simulink model "AircraftSim"  (R2025b)
settings: Solver=VariableStepAuto  StartTime=0.0  StopTime=10.0  RelTol=1e-3
libraries: simulink x6
settings Model: Creator=deepa  LastModifiedBy=deepa

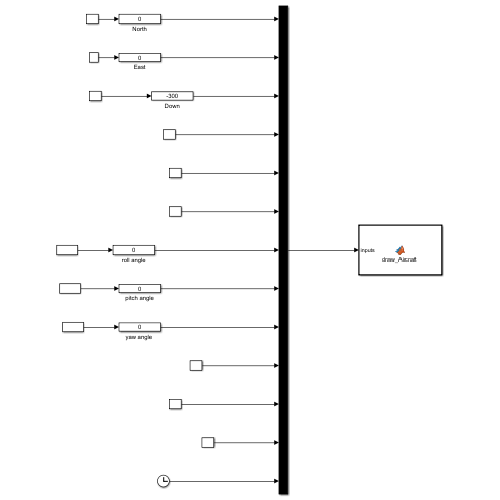
[thumbnail: Simulink's stored preview of the top-level diagram]
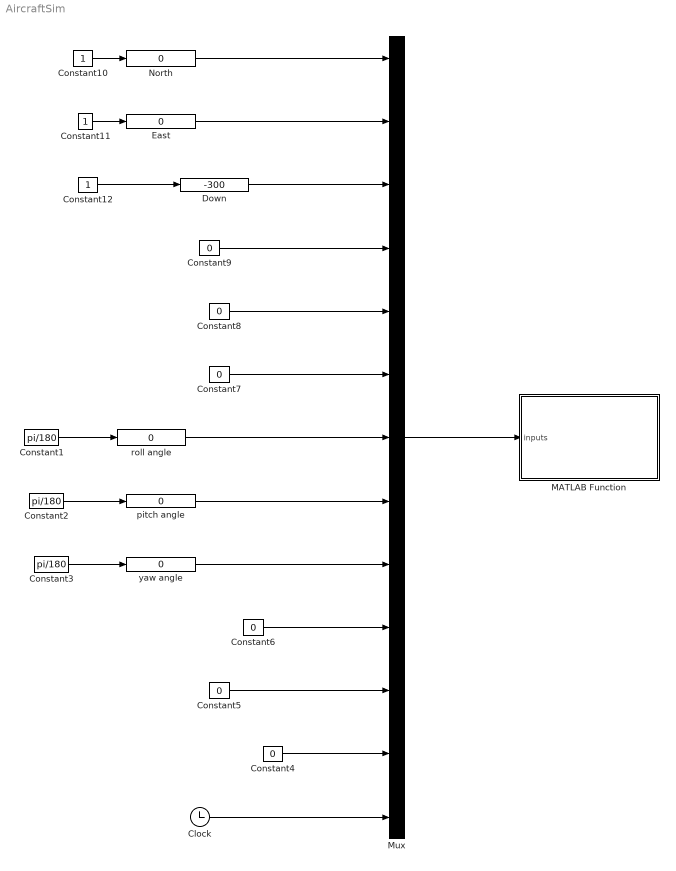
== system AircraftSim ==
  Clock : Clock
  Constant1 : Constant  Value=pi/180
  Constant10 : Constant
  Constant11 : Constant
  Constant12 : Constant
  Constant2 : Constant  Value=pi/180
  Constant3 : Constant  Value=pi/180
  Constant{4..9} (6 alike) : Constant  Value=0
  Down : simulink/Math Operations/Slider Gain  gain=-300  low=-1000  high=0
  East : simulink/Math Operations/Slider Gain  gain=0  low=-1000  high=1000
  MATLAB Function : MATLAB Function  TreatAsAtomicUnit=on
  Mux : Mux  Inputs=13
  North : simulink/Math Operations/Slider Gain  gain=0  low=-900  high=900
  pitch angle : simulink/Math Operations/Slider Gain  gain=0  low=-180  high=180
  roll angle : simulink/Math Operations/Slider Gain  gain=0  low=-180  high=180
  "yaw angle " : simulink/Math Operations/Slider Gain  gain=0  low=-180  high=180
  wires:
  Mux/1 -> MATLAB Function/1(inputs)
  roll angle/1 -> Mux/7
  pitch angle/1 -> Mux/8
  Constant2/1 -> pitch angle/1
  "yaw angle "/1 -> Mux/9
  Constant10/1 -> North/1
  North/1 -> Mux/1
  Constant11/1 -> East/1
  Constant12/1 -> Down/1
  East/1 -> Mux/2
  Constant1/1 -> roll angle/1
  Clock/1 -> Mux/13
  Constant3/1 -> "yaw angle "/1
  Constant4/1 -> Mux/12
  Constant5/1 -> Mux/11
  Constant6/1 -> Mux/10
  Constant7/1 -> Mux/6
  Constant8/1 -> Mux/5
  Constant9/1 -> Mux/4
  Down/1 -> Mux/3

== matlab function AircraftSim/MATLAB Function ==
  data: inputs input

function draw_Aircraft(inputs)

    pn = inputs(1); % Inertial North Position
    pe = inputs(2); % INertial East Position
    pd = inputs(3); 

    u = inputs(4);
    v = inputs(5);
    w = inputs(6);

    phi = inputs(7);
    theta = inputs(8);
    psi = inputs(9);

    p = inputs(10);
    q = inputs(11);
    r = inputs(12);

    t = inputs(13);

    persistent aircraft_handle
    persistent Vertices
    persistent Faces
    persistent facecolors


    if t == 0
        figure(1), clf
        [Vertices, Faces, facecolors] = defineAircraftBody;
        aircraft_handle = drawAircraftBody(Vertices, Faces, facecolors, pn, pe, pd, phi, theta, psi, []);

        title('Aircraft');
        xlabel('East');
        ylabel('North');
        zlabel('Down');
        view(32, 47)
        axis([-10 10 -10 10 -10 10]);
        hold on
    else
        drawAircraftBody(Vertices, Faces, facecolors, pn, pe, pd, phi, thet, psi, aircraft_handle);
    end
end



function drawAircraftBody(V, F, patchcolors, pn, pe, pd, phi, theta, psi, handle)

    V = rotate(V',phi, theta, psi)';
    V = translate(V', pn, pe, pd)';

    R = [0 1 0; 1 0 0; 0 0 -1];

    V = R*V;

    if isempty(handle)
        handle = patch('Vertices', V, 'Faces', F, 'FaceVertexCData', patchcolors,'FaceColor', 'flat');
    else
        set(handle, 'Vertices', V);
        drawnow
    end

end

function XYZ = rotate(XYZ, phi, theta, psi)
R_roll = [1 0 0; 0 cos(phi) -sin(phi); 0 sin(phi) cos(phi)];
R_pitch = [cos(theta) 0 sin(theta); 0 1 0; -sin(theta) 0 cos(theta)];
R_yaw = [cos(psi) -sin(psi) 0; sin(psi) cos(psi) 0; 0 0 1];
R = R_yaw * R_pitch * R_roll;
XYZ = R*XYZ;
end

function XYZ = translate(XYZ, pn, pe, pd)
    XYZ = XYZ + repmat([pn;pe;pd], 1, size(XYZ, 2));
end

function [V,F,colors] = defineAircraftBody()

 % vertices
    nose = [0 0.5 0.5; 0 0.5 -0.5; 0 -0.5 -0.5; 0 -0.5 0.5; -1 0 0];
    fuselage = [4 0 0];
    wing = [1 -3 0; 1 3 0; 2 3 0; 2 -3 0];
    hor_stabilizer = [4 -1 0; 4 1 0; 4.6 -1 0; 4.6 1 0];
    ver_stabilizer = [4.6 0 0; 4 0 0; 4.6 0 1]; 
    V = [nose; fuselage; wing; hor_stabilizer; ver_stabilizer];

    % Faces
    nose_f = [1 2 3; 3 4 1; 1 5 4; 3 4 5; 3 2 5; 1 2 5];
    fuselage_f = [2 3 6; 3 4 6; 1 4 6; 1 2 6];
    wing_f = [7 8 9; 7 9 10];
    hor_stabilizer_f = [11 12 14; 11 14 13];
    ver_stabilizer_f = [15 16 17];
    F = [nose_f; fuselage_f; wing_f; hor_stabilizer_f; ver_stabilizer_f];

    % ColorData
    red = [1 0 0];
    blue = [0 0 1];
    magenta = [1 0 1];
    yellow = [1 1 0];
    colors = [red; red; red; red; red; red; blue; blue; blue; blue; magenta; magenta; yellow; yellow; yellow];
end
